simulink model "CarSim_GS_LQR_Compensation"  (R2019a)
settings: Solver=VariableStepAuto  StartTime=0.0  StopTime=60  RelTol=1e-3
values from neighbouring files (symbols this model uses):
  Area = 2.4    [CarLQR.m]    (also in SpeedControlWithIntegral.m)
  Cr = 0.01    [CarLQR.m]    (also in SpeedControlWithIntegral.m)
  Cv = 0.32    [CarLQR.m]    (also in SpeedControlWithIntegral.m)
  delay = 0.2    [CarLQR.m]    (also in SpeedControlWithIntegral.m)
  F = Fe(1)    [CarLQR.m]    (also in SpeedControlWithIntegral.m)
  g = 9.81    [CarLQR.m]    (also in SpeedControlWithIntegral.m)
  H = Fe(2)    [CarLQR.m]    (also in SpeedControlWithIntegral.m)
  m = 1400    [CarLQR.m]    (also in SpeedControlWithIntegral.m = 2037)
  rho = 1.3    [CarLQR.m]    (also in SpeedControlWithIntegral.m)
  tauAct = 0.1    [CarLQR.m]    (also in SpeedControlWithIntegral.m)
  u0 = 0.5*rho*Area*Cv*v0^2 + m*g*Cr    (= 378.9528)    [CarLQR.m]    (also in SpeedControlWithIntegral.m = 441.4425)
  v0 = 22    [CarLQR.m]    (also in SpeedControlWithIntegral.m)
undefined symbols (not defined in the file or in its folder): mNominal, timeCom
libraries: simulink x4
settings Model: Creator=DELL  LastModifiedBy=DELL

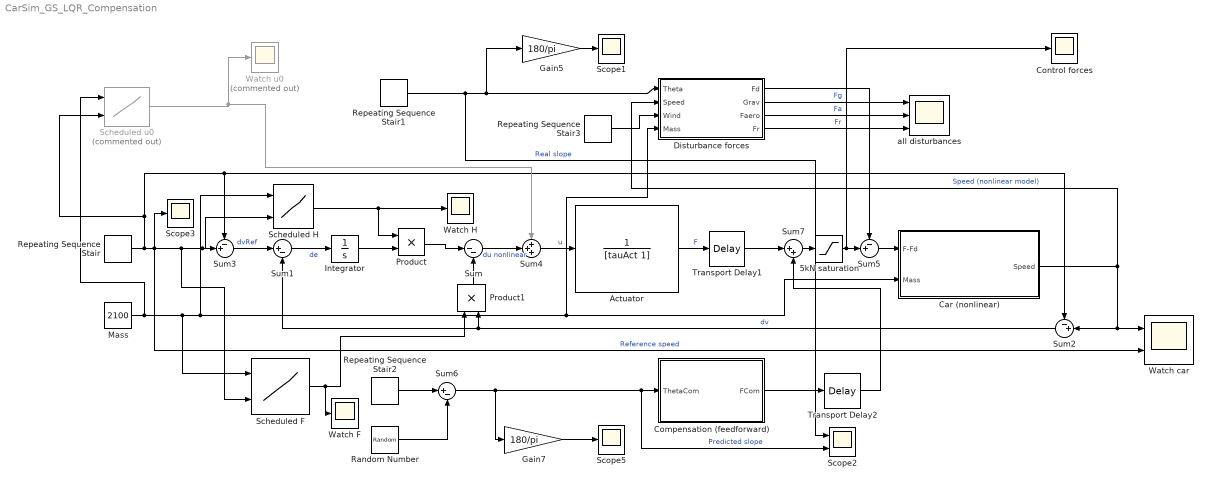
== system CarSim_GS_LQR_Compensation ==
  5kN saturation : Saturate  UpperLimit=5000  LowerLimit=-5000
  Actuator : TransferFcn  Denominator=[tauAct 1]
  Car (nonlinear) : Subsystem
  "Compensation (feedforward) " : Subsystem
  Control forces : Scope
  Disturbance forces : Subsystem
  Gain5 : Gain  Gain=180/pi
  Gain7 : Gain  Gain=180/pi
  Integrator : Integrator
  Mass : Constant  Value=2100
  Product : Product
  Product1 : Product
  Random Number : RandomNumber  Variance=0.000001  SampleTime=0.1
  Repeating Sequence Stair : simulink/Sources/Repeating Sequence Stair  OutValues=[23:1:28].'  tsamp=10  OutMin=[]  OutMax=[]  OutDataTypeStr=double  OutputDataTypeScalingMode=double  OutDataType=fixdt(0,8)  ConRadixGroup=Best Precision: Vector-wise  OutScaling=2^-12
  Repeating Sequence Stair1 : simulink/Sources/Repeating Sequence Stair  OutValues=[0.005 0.01 0 -0.005 -0.01].'  tsamp=0.5  OutMin=[]  OutMax=[]  OutDataTypeStr=double  OutputDataTypeScalingMode=double  OutDataType=fixdt(0,8)  ConRadixGroup=Best Precision: Vector-wise  OutScaling=2^-12
  Repeating Sequence Stair2 : simulink/Sources/Repeating Sequence Stair  OutValues=[0.005 0.01 0 -0.005 -0.01].'  tsamp=0.5  OutMin=[]  OutMax=[]  OutDataTypeStr=double  OutputDataTypeScalingMode=double  OutDataType=fixdt(0,8)  ConRadixGroup=Best Precision: Vector-wise  OutScaling=2^-12
  Repeating Sequence Stair3 : simulink/Sources/Repeating Sequence Stair  OutValues="[15 18  -15 -12 -18 12]/3.6.'"  tsamp=3  OutMin=[]  OutMax=[]  OutDataTypeStr=double  OutputDataTypeScalingMode=double  OutDataType=fixdt(0,8)  ConRadixGroup=Best Precision: Vector-wise  OutScaling=2^-12
  Scheduled F : Lookup_n-D  BreakpointsForDimension1=m  BreakpointsForDimension2=v0  Table=F  InternalRulePriority=Speed  RndMeth=Simplest  InputSameDT=on
  Scheduled H : Lookup_n-D  BreakpointsForDimension1=m  BreakpointsForDimension2=v0  Table=H  InternalRulePriority=Speed  RndMeth=Simplest  InputSameDT=on
  Scheduled u0 : Lookup_n-D  Commented=on  BreakpointsForDimension1=m  BreakpointsForDimension2=v0  Table=u0  InternalRulePriority=Speed  RndMeth=Simplest  InputSameDT=on
  Scope1 : Scope
  Scope2 : Scope  NumInputPorts=2
  Scope3 : Scope
  Scope5 : Scope
  Sum : Sum  Inputs=|--
  Sum1 : Sum  Inputs=|+-
  Sum2 : Sum  Inputs=-+|
  Sum3 : Sum  Inputs=-+|
  Sum4 : Sum  Inputs=+++
  Sum5 : Sum  Inputs=-+|
  Sum6 : Sum  Inputs=|+-
  Sum7 : Sum  Inputs=|++
  Transport Delay1 : TransportDelay  DelayTime=delay
  Transport Delay2 : TransportDelay  DelayTime=timeCom
  Watch F : Scope
  Watch H : Scope
  Watch car : Scope  NumInputPorts=2
  Watch u0 : Scope  Commented=on
  all disturbances : Scope  NumInputPorts=3
  wires:
  Gain7/1 -> Scope5/1
  Repeating Sequence Stair3/1 -> Disturbance forces/3(Wind)
  Repeating Sequence Stair2/1 -> Sum6/1
  Sum3/1 -> Sum1/1  "dvRef"
  Repeating Sequence Stair/1 -> Sum2/1, Sum3/1, Scheduled u0/2, Watch car/2, Scope3/1, Scheduled F/2, Scheduled H/2, Sum3/2  "Reference speed"
  Product/1 -> Sum/1
  Sum5/1 -> Car (nonlinear)/1("F-Fd ")
  Sum4/1 -> Actuator/1  "u"
  Sum1/1 -> Integrator/1  "de"
  Disturbance forces/2(Grav) -> all disturbances/1  "Fg"
  Disturbance forces/1(Fd) -> Sum5/1
  Product1/1 -> Sum/2
  Sum/1 -> Sum4/2  "du nonlinear"
  Car (nonlinear)/1(Speed) -> Disturbance forces/2(Speed), Watch car/1, Sum2/2  "Speed (nonlinear model)"
  Scheduled u0/1 -> Sum4/1, Watch u0/1
  Gain5/1 -> Scope1/1
  Disturbance forces/4(Fr) -> all disturbances/3  "Fr"
  Integrator/1 -> Product/2
  Sum2/1 -> Sum1/2, Product1/2  "dv"
  Disturbance forces/3(Faero) -> all disturbances/2  "Fa"
  Repeating Sequence Stair1/1 -> Scope2/1, Gain5/1, Disturbance forces/1(Theta)  "Real slope"
  Actuator/1 -> Transport Delay1/1  "F"
  Sum6/1 -> Scope2/2, "Compensation (feedforward) "/1(ThetaCom), Gain7/1  "Predicted slope"
  Random Number/1 -> Sum6/2
  "Compensation (feedforward) "/1(FCom) -> Transport Delay2/1
  Scheduled H/1 -> Watch H/1, Product/1
  Mass/1 -> Scheduled u0/1, Scheduled F/1, Disturbance forces/4(Mass), Car (nonlinear)/2(Mass), Scheduled H/1
  Scheduled F/1 -> Watch F/1, Product1/1
  Transport Delay1/1 -> Sum7/1
  Sum7/1 -> 5kN saturation/1
  5kN saturation/1 -> Control forces/1, Sum5/2
  Transport Delay2/1 -> Sum7/2

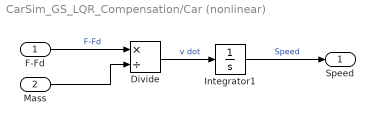
== system CarSim_GS_LQR_Compensation/Car (nonlinear) ==
  "F-Fd " : Inport
  Mass : Inport  Port=2
  Divide : Product  Inputs=*/
  Integrator1 : Integrator  InitialCondition=22
  Speed : Outport
  wires:
  Divide/1 -> Integrator1/1  "v dot"
  "F-Fd "/1 -> Divide/1  "F-Fd"
  Integrator1/1 -> Speed/1  "Speed"
  Mass/1 -> Divide/2

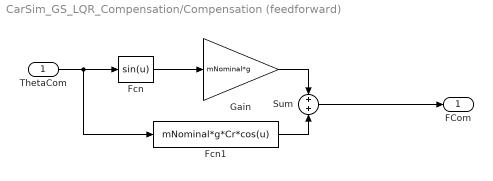
== system CarSim_GS_LQR_Compensation/Compensation (feedforward)  ==
  ThetaCom : Inport
  Fcn : Fcn  Expr=sin(u)
  Fcn1 : Fcn  Expr=mNominal*g*Cr*cos(u)
  Gain : Gain  Gain=mNominal*g
  Sum : Sum  Inputs=+|+
  FCom : Outport
  wires:
  ThetaCom/1 -> Fcn1/1, Fcn/1
  Gain/1 -> Sum/1
  Fcn1/1 -> Sum/2
  Fcn/1 -> Gain/1
  Sum/1 -> FCom/1

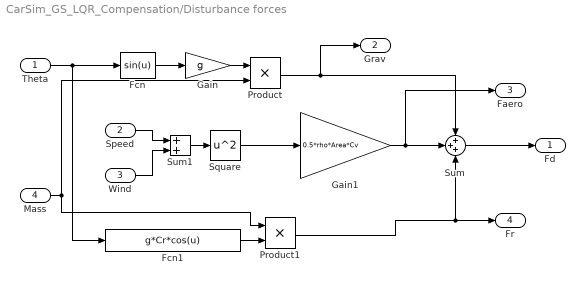
== system CarSim_GS_LQR_Compensation/Disturbance forces ==
  Theta : Inport
  Speed : Inport  Port=2
  Wind : Inport  Port=3
  Mass : Inport  Port=4
  Fcn : Fcn  Expr=sin(u)
  Fcn1 : Fcn  Expr=g*Cr*cos(u)
  Gain : Gain  Gain=g
  Gain1 : Gain  Gain=0.5*rho*Area*Cv
  Product : Product
  Product1 : Product
  Square : Math  Operator=square  SaturateOnIntegerOverflow=on
  Sum : Sum  Inputs=+++
  Sum1 : Sum
  Fd : Outport
  Grav : Outport  Port=2
  Faero : Outport  Port=3
  Fr : Outport  Port=4
  wires:
  Theta/1 -> Fcn1/1, Fcn/1
  Square/1 -> Gain1/1
  Gain1/1 -> Faero/1, Sum/2
  Sum/1 -> Fd/1
  Fcn/1 -> Gain/1
  Sum1/1 -> Square/1
  Speed/1 -> Sum1/1
  Wind/1 -> Sum1/2
  Product/1 -> Sum/1, Grav/1
  Gain/1 -> Product/1
  Mass/1 -> Product1/1, Product/2
  Fcn1/1 -> Product1/2
  Product1/1 -> Sum/3, Fr/1
